simulink model "First Exercise "  (R2018a)
settings: Solver=ode3  StartTime=0.0  StopTime=26  FixedStep=0.01  RelTol=1e-3
undefined symbols (not defined in the file): magnitude, w
settings Model: Creator=22132  LastModifiedBy=masouddayaghi
settings CodeAppCC: StateflowObjectComments=on

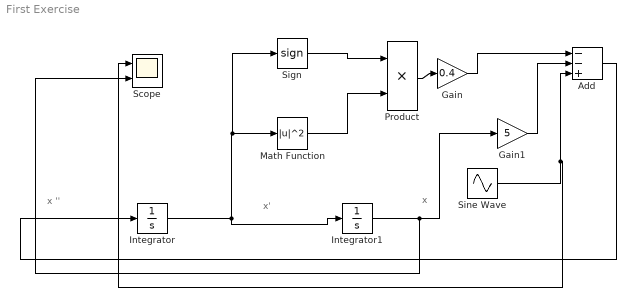
== system First Exercise  ==
  note: x
  note: x ''
  note: x'
  Add : Sum  Inputs=--+
  Gain : Gain  Gain=0.4
  Gain1 : Gain  Gain=5
  Integrator : Integrator
  Integrator1 : Integrator
  Math Function : Math  Operator=magnitude^2  OutputSignalType=real  SaturateOnIntegerOverflow=on
  Product : Product
  Scope : Scope  NumInputPorts=2
  Sign : Signum
  Sine Wave : Sin  Frequency=w  SampleTime=0
  wires:
  Integrator/1 -> Sign/1, Math Function/1, Integrator1/1
  Product/1 -> Gain/1
  Integrator1/1 -> Scope/2, Gain1/1
  Gain1/1 -> Add/2
  Gain/1 -> Add/1
  Sign/1 -> Product/1
  Math Function/1 -> Product/2
  Sine Wave/1 -> Scope/1, Add/3
  Add/1 -> Integrator/1
